simulink model "signal_conversion"  (R2020b)
settings: Solver=VariableStepAuto  StartTime=0.0  StopTime=10.0  RelTol=1e-3
settings Model: Creator=conno  LastModifiedBy=conno

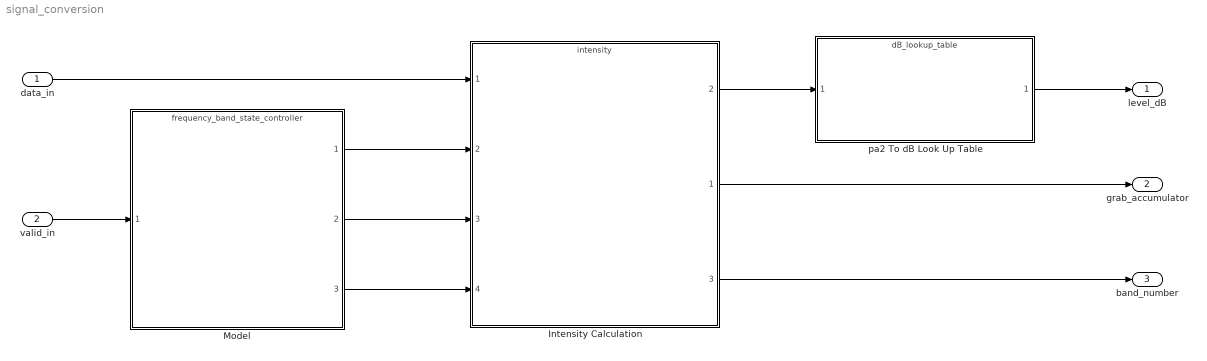
== system signal_conversion ==
  data_in : Inport
  valid_in : Inport  Port=2
  Intensity Calculation : ModelReference  ModelNameDialog=intensity.slx  SimulationMode=Normal  ModelReferenceVersion=2.35
      settings: PortSchema="{\"entries\":[{\"content\":{\"sides\":[{\"content\":{\"connectorIds\":[\"In1\",\"In2\",\"In3\",\"In4\"]},\"type\":\"ConnectorPlacement.EquallySpacedRectSide\",\"uuid\":\"1715ac82-9bf9-45f0-89dd-ef254743e0d0\"},{\"content\":{\"connectorIds\":[\"Out2\",\"Out1\",\"Out3\"],\"side\":\"RIGHT\"},\"type\":\"ConnectorPlacement.EquallySpacedRectSide\",\"uuid\":\"1ac9df1c-3178-4a7b-9102-20b65dc3805c\"},{\"content\":{\"connectorIds\":[],\"side\":\"TOP\"},\"type\":\"ConnectorPlacement.EquallySpacedRectSide\",\"uuid\":\"25569bb4-aab4-4363-9b28-b47c18a3e185\"},{\"content\":{\"connectorIds\":[],\"side\":\"HIDDEN\"},\"type\":\"ConnectorPlacement.EquallySpacedRectSide\",\"uuid\":\"29078c1d-30f1-4610-ae90-b869cbef1c5f\"}]},\"type\":\"ConnectorPlacement.EquallySpacedConnector\",\"uuid\":\"9fe03e1d-ee03-41fe-8a8f-68791f98f5c0\"}],\"packageUris\":[\"http://schema.mathworks.com/mf0/Connector/R2020b\"],\"version\":\"1.0\"}"
  Model : ModelReference  ModelNameDialog=frequency_band_state_controller.slx  SimulationMode=Normal  ModelReferenceVersion=2.31
  pa2 To dB Look Up Table : ModelReference  ModelNameDialog=dB_lookup_table.slx  SimulationMode=Normal  ModelReferenceVersion=2.31
  level_dB : Outport
  grab_accumulator : Outport  Port=2
  band_number : Outport  Port=3
  wires:
  pa2 To dB Look Up Table/1 -> level_dB/1
  Intensity Calculation/2 -> pa2 To dB Look Up Table/1
  Intensity Calculation/1 -> grab_accumulator/1
  Intensity Calculation/3 -> band_number/1
  Model/1 -> Intensity Calculation/2
  Model/2 -> Intensity Calculation/3
  Model/3 -> Intensity Calculation/4
  valid_in/1 -> Model/1
  data_in/1 -> Intensity Calculation/1
